simulink model "cf_compare_model"  (R2016a)
settings: Solver=FixedStepAuto  StartTime=0.0  StopTime=50  FixedStep=dt  RelTol=1e-3
values from neighbouring files (symbols this model uses):
  circ_amp = 3    [cf_pid_compare.m]
  circ_w = k    (= 0.666666666667)    [cf_pid_compare.m]
  ic = [-3 0 0 0 0 0 0 0 0 0 0 0]    [cf_pid_compare.m]    (also in main.m = [0 0 0 0 0 0 0 0 0 0 0 0])
  r2d = 180/pi    (= 57.2957795131)    [main.m]
  x_init = 0.0    (= 0)    [cf_pid_compare.m]
  x_vel = 1.0    (= 1)    [cf_pid_compare.m]
undefined symbols (not defined in the file or in its folder): default_ctl, est, geometric_ctl, pid_ctl
undefined symbols (not defined in the file): cf2
libraries: simulink x18, vrlib x12, aerolibtransform2 x12, cstblocks x8, aerolibutil x6, aerolibnav x3, dspmathops x2
(part 2 of 2)

== system cf_compare_model/Vehicle1/PWM 2 Speed ==
  PWM : Inport
  Add{,1..3} (4 alike) : Sum
  Constant{,1..3} (4 alike) : Constant  Value=model.pwm_offset
  Demux : Demux
  Gain{,1..3} (4 alike) : Gain  Gain=model.pwm_gain
  Mux : Mux
  Omega : Outport
  wires:
  Add3/1 -> Mux/4
  Demux/4 -> Gain3/1
  Add2/1 -> Mux/3
  Demux/3 -> Gain2/1
  Add1/1 -> Mux/2
  Demux/2 -> Gain1/1
  Constant3/1 -> Add3/1
  Gain3/1 -> Add3/2
  Constant2/1 -> Add2/1
  Gain2/1 -> Add2/2
  Constant1/1 -> Add1/1
  Gain1/1 -> Add1/2
  Add/1 -> Mux/1
  Demux/1 -> Gain/1
  Mux/1 -> Omega/1
  PWM/1 -> Demux/1
  Constant/1 -> Add/1
  Gain/1 -> Add/2

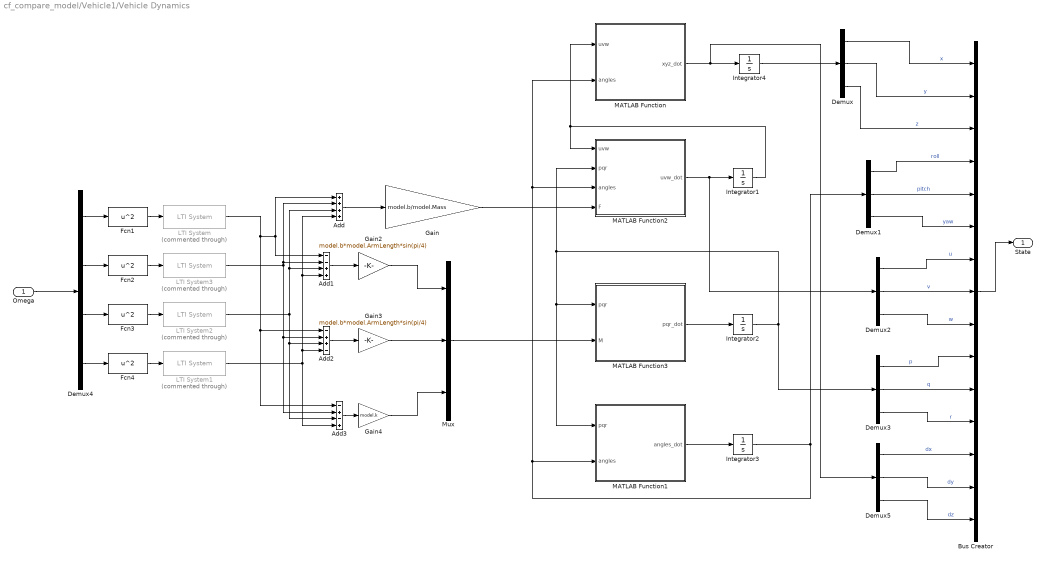
== system cf_compare_model/Vehicle1/Vehicle Dynamics ==
  Omega : Inport
  Add : Sum  Inputs=++++
  Add1 : Sum  Inputs=--++
  Add2 : Sum  Inputs=-++-
  Add3 : Sum  Inputs=-+-+
  Bus Creator : BusCreator  Inputs='x','y','z','roll','pitch','yaw','u','v','w','p','q','r','dx','dy','dz'
  Demux{,1..3,5} (5 alike) : Demux  Outputs=3
  Demux4 : Demux
  Fcn{1..4} (4 alike) : Fcn  Expr=u^2
  Gain : Gain  Gain=model.b/model.Mass
  Gain2 : Gain  Gain=model.b*model.ArmLength*sin(pi/4)
  Gain3 : Gain  Gain=model.b*model.ArmLength*sin(pi/4)
  Gain4 : Gain  Gain=model.k
  Integrator1 : Integrator  InitialCondition=ic(7:9)
  Integrator2 : Integrator  InitialCondition=ic(10:12)
  Integrator3 : Integrator  InitialCondition=ic(4:6)
  Integrator4 : Integrator  InitialCondition=ic(1:3)
  LTI System{,1..3} (4 alike) : cstblocks/LTI System  Commented=through  sys=model.motorDyn  IC=[]
  MATLAB Function : MATLAB Function  TreatAsAtomicUnit=on
  MATLAB Function1 : MATLAB Function  TreatAsAtomicUnit=on
  MATLAB Function2 : MATLAB Function  TreatAsAtomicUnit=on
  MATLAB Function3 : MATLAB Function  TreatAsAtomicUnit=on
  Mux : Mux  Inputs=3
  State : Outport
  wires:
  Omega/1 -> Demux4/1
  Demux4/4 -> Fcn4/1
  Demux4/3 -> Fcn3/1
  Demux4/2 -> Fcn2/1
  Demux4/1 -> Fcn1/1
  Demux2/2 -> Bus Creator/8  "v"
  Demux1/2 -> Bus Creator/5  "pitch"
  Demux3/1 -> Bus Creator/10  "p"
  Demux3/2 -> Bus Creator/11  "q"
  Demux3/3 -> Bus Creator/12  "r"
  Demux2/3 -> Bus Creator/9  "w"
  Demux2/1 -> Bus Creator/7  "u"
  Demux1/1 -> Bus Creator/4  "roll"
  Demux1/3 -> Bus Creator/6  "yaw"
  Demux/3 -> Bus Creator/3  "z"
  Demux/2 -> Bus Creator/2  "y"
  Demux/1 -> Bus Creator/1  "x"
  Integrator4/1 -> Demux/1
  Integrator2/1 -> MATLAB Function3/1(pqr), MATLAB Function1/1(pqr), MATLAB Function2/2(pqr), Demux3/1
  Integrator1/1 -> MATLAB Function2/1(uvw), MATLAB Function/1(uvw)
  Integrator3/1 -> MATLAB Function1/2(angles), MATLAB Function2/3(angles), MATLAB Function/2(angles), Demux1/1
  MATLAB Function1/1(angles_dot) -> Integrator3/1
  MATLAB Function3/1(pqr_dot) -> Integrator2/1
  MATLAB Function2/1(uvw_dot) -> Demux2/1, Integrator1/1
  MATLAB Function/1(xyz_dot) -> Integrator4/1, Demux5/1
  Mux/1 -> MATLAB Function3/2(M)
  Gain/1 -> MATLAB Function2/4(F)
  Gain3/1 -> Mux/2
  Add3/1 -> Gain4/1
  Gain4/1 -> Mux/3
  Gain2/1 -> Mux/1
  Add2/1 -> Gain3/1
  Add1/1 -> Gain2/1
  Bus Creator/1 -> State/1
  Fcn1/1 -> LTI System/1
  Fcn2/1 -> LTI System3/1
  Fcn3/1 -> LTI System2/1
  Fcn4/1 -> LTI System1/1
  Add/1 -> Gain/1
  LTI System1/1 -> Add3/4, Add2/4, Add1/4, Add/4
  LTI System2/1 -> Add3/3, Add2/3, Add/3, Add1/3
  LTI System3/1 -> Add3/2, Add2/2, Add/2, Add1/2
  LTI System/1 -> Add3/1, Add2/1, Add1/1, Add/1
  Demux5/1 -> Bus Creator/13  "dx"
  Demux5/2 -> Bus Creator/14  "dy"
  Demux5/3 -> Bus Creator/15  "dz"

== system cf_compare_model/Vehicle3/PWM 2 Speed ==
  PWM : Inport
  Add{,1..3} (4 alike) : Sum
  Constant{,1..3} (4 alike) : Constant  Value=model.pwm_offset
  Demux : Demux
  Gain{,1..3} (4 alike) : Gain  Gain=model.pwm_gain
  Mux : Mux
  Omega : Outport
  wires:
  Add3/1 -> Mux/4
  Demux/4 -> Gain3/1
  Add2/1 -> Mux/3
  Demux/3 -> Gain2/1
  Add1/1 -> Mux/2
  Demux/2 -> Gain1/1
  Constant3/1 -> Add3/1
  Gain3/1 -> Add3/2
  Constant2/1 -> Add2/1
  Gain2/1 -> Add2/2
  Constant1/1 -> Add1/1
  Gain1/1 -> Add1/2
  Add/1 -> Mux/1
  Demux/1 -> Gain/1
  Mux/1 -> Omega/1
  PWM/1 -> Demux/1
  Constant/1 -> Add/1
  Gain/1 -> Add/2

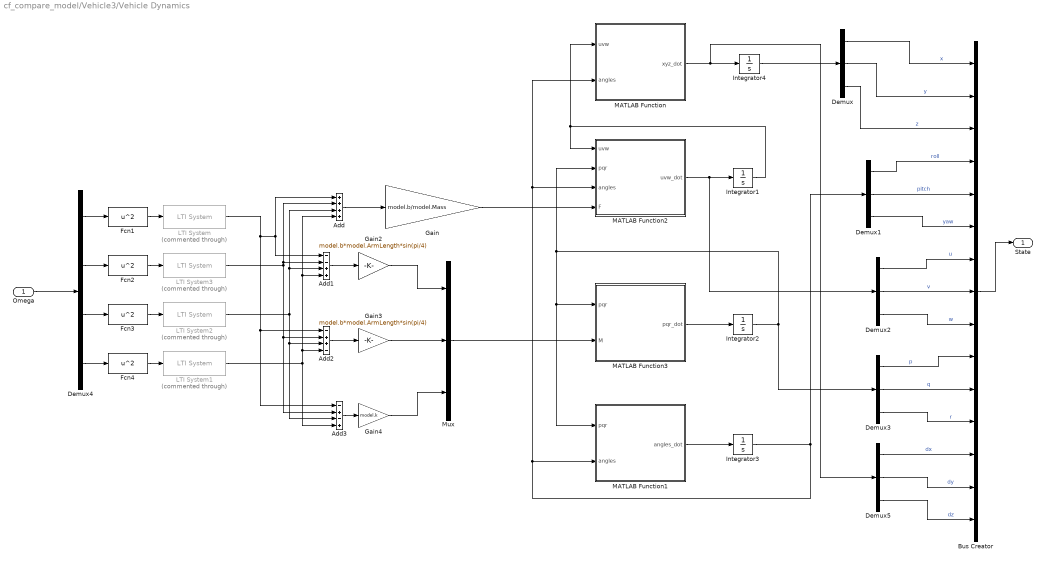
== system cf_compare_model/Vehicle3/Vehicle Dynamics ==
  Omega : Inport
  Add : Sum  Inputs=++++
  Add1 : Sum  Inputs=--++
  Add2 : Sum  Inputs=-++-
  Add3 : Sum  Inputs=-+-+
  Bus Creator : BusCreator  Inputs='x','y','z','roll','pitch','yaw','u','v','w','p','q','r','dx','dy','dz'
  Demux{,1..3,5} (5 alike) : Demux  Outputs=3
  Demux4 : Demux
  Fcn{1..4} (4 alike) : Fcn  Expr=u^2
  Gain : Gain  Gain=model.b/model.Mass
  Gain2 : Gain  Gain=model.b*model.ArmLength*sin(pi/4)
  Gain3 : Gain  Gain=model.b*model.ArmLength*sin(pi/4)
  Gain4 : Gain  Gain=model.k
  Integrator1 : Integrator  InitialCondition=ic(7:9)
  Integrator2 : Integrator  InitialCondition=ic(10:12)
  Integrator3 : Integrator  InitialCondition=ic(4:6)
  Integrator4 : Integrator  InitialCondition=ic(1:3)
  LTI System{,1..3} (4 alike) : cstblocks/LTI System  Commented=through  sys=model.motorDyn  IC=[]
  MATLAB Function : MATLAB Function  TreatAsAtomicUnit=on
  MATLAB Function1 : MATLAB Function  TreatAsAtomicUnit=on
  MATLAB Function2 : MATLAB Function  TreatAsAtomicUnit=on
  MATLAB Function3 : MATLAB Function  TreatAsAtomicUnit=on
  Mux : Mux  Inputs=3
  State : Outport
  wires:
  Omega/1 -> Demux4/1
  Demux4/4 -> Fcn4/1
  Demux4/3 -> Fcn3/1
  Demux4/2 -> Fcn2/1
  Demux4/1 -> Fcn1/1
  Demux2/2 -> Bus Creator/8  "v"
  Demux1/2 -> Bus Creator/5  "pitch"
  Demux3/1 -> Bus Creator/10  "p"
  Demux3/2 -> Bus Creator/11  "q"
  Demux3/3 -> Bus Creator/12  "r"
  Demux2/3 -> Bus Creator/9  "w"
  Demux2/1 -> Bus Creator/7  "u"
  Demux1/1 -> Bus Creator/4  "roll"
  Demux1/3 -> Bus Creator/6  "yaw"
  Demux/3 -> Bus Creator/3  "z"
  Demux/2 -> Bus Creator/2  "y"
  Demux/1 -> Bus Creator/1  "x"
  Integrator4/1 -> Demux/1
  Integrator2/1 -> MATLAB Function3/1(pqr), MATLAB Function1/1(pqr), MATLAB Function2/2(pqr), Demux3/1
  Integrator1/1 -> MATLAB Function2/1(uvw), MATLAB Function/1(uvw)
  Integrator3/1 -> MATLAB Function1/2(angles), MATLAB Function2/3(angles), MATLAB Function/2(angles), Demux1/1
  MATLAB Function1/1(angles_dot) -> Integrator3/1
  MATLAB Function3/1(pqr_dot) -> Integrator2/1
  MATLAB Function2/1(uvw_dot) -> Demux2/1, Integrator1/1
  MATLAB Function/1(xyz_dot) -> Integrator4/1, Demux5/1
  Mux/1 -> MATLAB Function3/2(M)
  Gain/1 -> MATLAB Function2/4(F)
  Gain3/1 -> Mux/2
  Add3/1 -> Gain4/1
  Gain4/1 -> Mux/3
  Gain2/1 -> Mux/1
  Add2/1 -> Gain3/1
  Add1/1 -> Gain2/1
  Bus Creator/1 -> State/1
  Fcn1/1 -> LTI System/1
  Fcn2/1 -> LTI System3/1
  Fcn3/1 -> LTI System2/1
  Fcn4/1 -> LTI System1/1
  Add/1 -> Gain/1
  LTI System1/1 -> Add3/4, Add2/4, Add1/4, Add/4
  LTI System2/1 -> Add3/3, Add2/3, Add/3, Add1/3
  LTI System3/1 -> Add3/2, Add2/2, Add/2, Add1/2
  LTI System/1 -> Add3/1, Add2/1, Add1/1, Add/1
  Demux5/1 -> Bus Creator/13  "dx"
  Demux5/2 -> Bus Creator/14  "dy"
  Demux5/3 -> Bus Creator/15  "dz"

== system cf_compare_model/circle xy/acc_circ ==
  Constant : Constant  Value=0
  Mux : Mux  Inputs=3
  Sine Wave1 : Sin  Amplitude=circ_amp*circ_w^2  Frequency=circ_w  Phase=3*pi/2  SampleTime=0
  Sine Wave2 : Sin  Amplitude=circ_amp*circ_w^2  Frequency=circ_w  Phase=pi  SampleTime=0
  Acc : Outport
  wires:
  Sine Wave2/1 -> Mux/3
  Constant/1 -> Mux/1
  Sine Wave1/1 -> Mux/2
  Mux/1 -> Acc/1

== system cf_compare_model/circle xy/jerk_circ ==
  Constant : Constant  Value=0
  Mux : Mux  Inputs=3
  Sine Wave1 : Sin  Amplitude=circ_amp*circ_w^3  Frequency=circ_w  SampleTime=0
  Sine Wave2 : Sin  Amplitude=circ_amp*circ_w^3  Frequency=circ_w  Phase=3*pi/2  SampleTime=0
  Jerk : Outport
  wires:
  Sine Wave2/1 -> Mux/3
  Constant/1 -> Mux/1
  Sine Wave1/1 -> Mux/2
  Mux/1 -> Jerk/1

== system cf_compare_model/circle xy/snap_circ ==
  Constant : Constant  Value=0
  Mux : Mux  Inputs=3
  Sine Wave1 : Sin  Amplitude=circ_amp*circ_w^4  Frequency=circ_w  Phase=pi/2  SampleTime=0
  Sine Wave2 : Sin  Amplitude=circ_amp*circ_w^4  Frequency=circ_w  SampleTime=0
  Snap : Outport
  wires:
  Sine Wave2/1 -> Mux/3
  Constant/1 -> Mux/1
  Sine Wave1/1 -> Mux/2
  Mux/1 -> Snap/1

== system cf_compare_model/circle xy/vel_circ ==
  Constant : Constant  Value=x_vel
  Mux : Mux  Inputs=3
  Sine Wave1 : Sin  Amplitude=circ_amp*circ_w  Frequency=circ_w  Phase=pi  SampleTime=0
  Sine Wave2 : Sin  Amplitude=circ_amp*circ_w  Frequency=circ_w  Phase=pi/2  SampleTime=0
  Vel : Outport
  wires:
  Sine Wave2/1 -> Mux/3
  Constant/1 -> Mux/1
  Sine Wave1/1 -> Mux/2
  Mux/1 -> Vel/1

== system cf_compare_model/circle yz /acc_circ ==
  Constant : Constant  Value=0
  Mux : Mux  Inputs=3
  Sine Wave1 : Sin  Amplitude=circ_amp*circ_w^2  Frequency=circ_w  Phase=3*pi/2  SampleTime=0
  Sine Wave2 : Sin  Amplitude=circ_amp*circ_w^2  Frequency=circ_w  Phase=pi  SampleTime=0
  Acc : Outport
  wires:
  Sine Wave2/1 -> Mux/3
  Constant/1 -> Mux/1
  Sine Wave1/1 -> Mux/2
  Mux/1 -> Acc/1

== system cf_compare_model/circle yz /jerk_circ ==
  Constant : Constant  Value=0
  Mux : Mux  Inputs=3
  Sine Wave1 : Sin  Amplitude=circ_amp*circ_w^3  Frequency=circ_w  SampleTime=0
  Sine Wave2 : Sin  Amplitude=circ_amp*circ_w^3  Frequency=circ_w  Phase=3*pi/2  SampleTime=0
  Jerk : Outport
  wires:
  Sine Wave2/1 -> Mux/3
  Constant/1 -> Mux/1
  Sine Wave1/1 -> Mux/2
  Mux/1 -> Jerk/1

== system cf_compare_model/circle yz /snap_circ ==
  Constant : Constant  Value=0
  Mux : Mux  Inputs=3
  Sine Wave1 : Sin  Amplitude=circ_amp*circ_w^4  Frequency=circ_w  Phase=pi/2  SampleTime=0
  Sine Wave2 : Sin  Amplitude=circ_amp*circ_w^4  Frequency=circ_w  SampleTime=0
  Snap : Outport
  wires:
  Sine Wave2/1 -> Mux/3
  Constant/1 -> Mux/1
  Sine Wave1/1 -> Mux/2
  Mux/1 -> Snap/1

== system cf_compare_model/circle yz /vel_circ ==
  Constant : Constant  Value=x_vel
  Mux : Mux  Inputs=3
  Sine Wave1 : Sin  Amplitude=circ_amp*circ_w  Frequency=circ_w  Phase=pi  SampleTime=0
  Sine Wave2 : Sin  Amplitude=circ_amp*circ_w  Frequency=circ_w  Phase=pi/2  SampleTime=0
  Vel : Outport
  wires:
  Sine Wave2/1 -> Mux/3
  Constant/1 -> Mux/1
  Sine Wave1/1 -> Mux/2
  Mux/1 -> Vel/1

== system cf_compare_model/PID/Estimator/AddNoise1 ==
  Signal : Inport
  AddNoise : Subsystem
  AddNoise1 : Subsystem
  AddNoise2 : Subsystem
  Demux : Demux  Outputs=3
  Mux : Mux  Inputs=3
  +Noise : Outport
  wires:
  Mux/1 -> +Noise/1
  Signal/1 -> Demux/1
  AddNoise2/1(+Noise) -> Mux/3
  AddNoise1/1(+Noise) -> Mux/2
  AddNoise/1(+Noise) -> Mux/1
  Demux/1 -> AddNoise/1(Signal)
  Demux/3 -> AddNoise2/1(Signal)
  Demux/2 -> AddNoise1/1(Signal)

== system cf_compare_model/PID/Estimator/AddNoise3 ==
  Signal : Inport
  AddNoise : Subsystem
  AddNoise1 : Subsystem
  AddNoise2 : Subsystem
  Demux : Demux  Outputs=3
  Mux : Mux  Inputs=3
  +Noise : Outport
  wires:
  Demux/2 -> AddNoise1/1(Signal)
  Demux/3 -> AddNoise2/1(Signal)
  Demux/1 -> AddNoise/1(Signal)
  AddNoise/1(+Noise) -> Mux/1
  AddNoise1/1(+Noise) -> Mux/2
  AddNoise2/1(+Noise) -> Mux/3
  Signal/1 -> Demux/1
  Mux/1 -> +Noise/1

== system cf_compare_model/PID/Estimator/Mahoney ==
  A : Inport  PortDimensions=[1 3]
  ω : Inport  Port=2  PortDimensions=[1 3]
  Vicon : Inport  Port=3
  q : Inport  Port=4  PortDimensions=[1 4]
  Acceleration Error Estimate : Scope
  Add : Sum  Inputs=+++
  Add1 : Sum
  Constant : Constant  Value=0
  Cross Product : vrlib/Utilities/Cross Product
  Cross Product1 : vrlib/Utilities/Cross Product
  Gain1 : Gain  Gain=0.5
  Integrator : Integrator
  Integrator1 : Integrator  InitialCondition=[1,0,0,0]
  Ki : Gain  Gain=est.Ki
  Kp : Gain  Gain=est.Kp
  Mux : Mux  Inputs=2
  Normalize Vector : vrlib/Utilities/Normalize Vector  maxzero=.01
  Normalize Vector1 : vrlib/Utilities/Normalize Vector  maxzero=10e-4
  Total Error Estimate : Scope
  Vicon Error Estimate : Scope
  calc v : MATLAB Function  TreatAsAtomicUnit=on
  calc v3 : MATLAB Function  TreatAsAtomicUnit=on
  quatprod : MATLAB Function  TreatAsAtomicUnit=on
  Quaternion : Outport
  wires:
  A/1 -> Normalize Vector/1
  Constant/1 -> Mux/1
  Add1/1 -> Integrator/1, Kp/1, Total Error Estimate/1
  Ki/1 -> Add/2
  calc v/1(v) -> Cross Product/1, Cross Product1/2
  Add/1 -> Mux/2
  Kp/1 -> Add/1
  Gain1/1 -> Integrator1/1
  quatprod/1(ab) -> Gain1/1
  Mux/1 -> quatprod/2(b)
  Integrator/1 -> Ki/1
  Integrator1/1 -> Normalize Vector1/1
  Normalize Vector1/1 -> Quaternion/1
  q/1 -> calc v/1(q), quatprod/1(a)
  Cross Product/1 -> Acceleration Error Estimate/1, Add1/2
  Vicon/1 -> calc v3/1(q)
  Cross Product1/1 -> Vicon Error Estimate/1, Add1/1
  calc v3/1(v) -> Cross Product1/1
  Normalize Vector/1 -> Cross Product/2
  ω/1 -> Add/3

== system cf_compare_model/PID/PID Controller/Attitude Control ==
  desired_attitude : Inport
  attitutde : Inport  Port=2
  Demux : Demux  Outputs=3
  Demux1 : Demux  Outputs=3
  Gain : Gain  Gain=r2d
  Gain1 : Gain  Gain=r2d
  Gain2 : Gain  Gain=r2d
  Mux : Mux  Inputs=3
  PID : Subsystem
  PID1 : Subsystem
  PID2 : Subsystem
  Saturation : Saturate  UpperLimit=sat(3)  LowerLimit=-sat(3)
  Saturation1 : Saturate  UpperLimit=sat(2)  LowerLimit=-sat(2)
  Saturation2 : Saturate  UpperLimit=sat(1)  LowerLimit=-sat(1)
  desired_rates : Outport
  wires:
  [pitch] -> PID1/2(Measured)
  [desired_pitch] -> PID1/1(Desired)
  [desired_roll] -> PID/1(Desired)
  [roll] -> PID/2(Measured)
  desired_attitude/1 -> Demux/1
  Demux/1 -> Saturation2/1
  Demux/2 -> Saturation1/1
  Demux/3 -> [desired_yaw]
  attitutde/1 -> Demux1/1
  Demux1/1 -> Gain/1
  Demux1/2 -> Gain1/1
  Demux1/3 -> Gain2/1
  [yaw] -> PID2/2(Measured)
  Gain/1 -> [roll]
  Gain1/1 -> [pitch]
  Gain2/1 -> [yaw]
  [desired_yaw] -> PID2/1(Desired)
  PID/1(Output) -> Mux/1
  PID2/1(Output) -> Saturation/1
  PID1/1(Output) -> Mux/2
  Mux/1 -> desired_rates/1
  Saturation/1 -> Mux/3
  Saturation1/1 -> [desired_pitch]
  Saturation2/1 -> [desired_roll]

== system cf_compare_model/PID/PID Controller/Linear Velocity Control ==
  note: ROLL CONTROLS Y TRANSLATION
  note: PITCH CONTROLS X TRANSLATION
  position_error : Inport
  velocity : Inport  Port=2
  Add : Sum
  Demux : Demux  Outputs=3
  Demux1 : Demux  Outputs=3
  "Min_thrust " : Constant  Value=default_ctl.pwm  SampleTime=0
  Mux : Mux  Inputs=2
  PID : Subsystem
  PID1 : Subsystem
  PID_Altitude : Subsystem
  Saturation2 : Saturate  UpperLimit=default_ctl.sat(4,1)  LowerLimit=0
  Scope : Scope
  Terminator : Terminator
  desired_attitude : Outport
  desired_thrust : Outport  Port=2
  wires:
  [y_e] -> PID/1(Desired)
  Saturation2/1 -> Scope/1, desired_thrust/1
  "Min_thrust "/1 -> Add/2
  Add/1 -> Saturation2/1
  PID_Altitude/1(Adjust) -> Add/1
  position_error/1 -> Demux/1
  Demux/1 -> [x_e]
  Demux/2 -> [y_e]
  Demux/3 -> [z_e]
  [z_e] -> PID_Altitude/1(z_error)
  velocity/1 -> Demux1/1
  Demux1/1 -> [v_x]
  Demux1/2 -> [v_y]
  Demux1/3 -> Terminator/1
  [v_y] -> PID/2(Measured)
  Mux/1 -> desired_attitude/1
  PID/1(Output) -> Mux/1
  [x_e] -> PID1/1(Desired)
  [v_x] -> PID1/2(Measured)
  PID1/1(Output) -> Mux/2

== system cf_compare_model/PID/PID Controller/Motor Mix ==
  rpy : Inport
  T : Inport  Port=2
  Constant : Constant  Value=mix
  Demux : Demux  Outputs=3
  Mux : Mux
  Product : Product  Multiplication=Matrix(*)
  PWM : Outport
  wires:
  T/1 -> Mux/4
  Mux/1 -> Product/2
  Product/1 -> PWM/1
  Constant/1 -> Product/1
  rpy/1 -> Demux/1
  Demux/2 -> Mux/2
  Demux/1 -> Mux/1
  Demux/3 -> Mux/3

== system cf_compare_model/PID/PID Controller/Rate Control ==
  note: roll
      | pitch
      | yaw
  desired_rates : Inport
  rates : Inport  Port=2
  Demux : Demux  Outputs=3
  Demux1 : Demux  Outputs=3
  Gain : Gain  Gain=r2d
  Gain1 : Gain  Gain=r2d
  Gain2 : Gain  Gain=r2d
  Mux : Mux  Inputs=3
  PID : Subsystem
  PID1 : Subsystem
  PID2 : Subsystem
  rpy_cmd : Outport
  wires:
  desired_rates/1 -> Demux/1
  Demux/1 -> [desired_droll]
  Demux/2 -> [desired_dpitch]
  Demux/3 -> [desired_dyaw]
  rates/1 -> Demux1/1
  Demux1/1 -> Gain/1
  Demux1/2 -> Gain1/1
  Demux1/3 -> Gain2/1
  Gain/1 -> [droll]
  Gain1/1 -> [dpitch]
  Gain2/1 -> [dyaw]
  PID2/1(Output) -> Mux/3
  PID1/1(Output) -> Mux/2
  PID/1(Output) -> Mux/1
  Mux/1 -> rpy_cmd/1
  [desired_dyaw] -> PID2/1(Desired)
  [desired_droll] -> PID/1(Desired)
  [desired_dpitch] -> PID1/1(Desired)
  [dpitch] -> PID1/2(Measured)
  [droll] -> PID/2(Measured)
  [dyaw] -> PID2/2(Measured)

== system cf_compare_model/PID/Vehicle/PWM 2 Speed ==
  PWM : Inport
  Add{,1..3} (4 alike) : Sum
  Constant{,1..3} (4 alike) : Constant  Value=model.pwm_offset
  Demux : Demux
  Gain{,1..3} (4 alike) : Gain  Gain=model.pwm_gain
  Mux : Mux
  Omega : Outport
  wires:
  Gain/1 -> Add/2
  Constant/1 -> Add/1
  PWM/1 -> Demux/1
  Mux/1 -> Omega/1
  Demux/1 -> Gain/1
  Add/1 -> Mux/1
  Gain1/1 -> Add1/2
  Constant1/1 -> Add1/1
  Gain2/1 -> Add2/2
  Constant2/1 -> Add2/1
  Gain3/1 -> Add3/2
  Constant3/1 -> Add3/1
  Demux/2 -> Gain1/1
  Add1/1 -> Mux/2
  Demux/3 -> Gain2/1
  Add2/1 -> Mux/3
  Demux/4 -> Gain3/1
  Add3/1 -> Mux/4

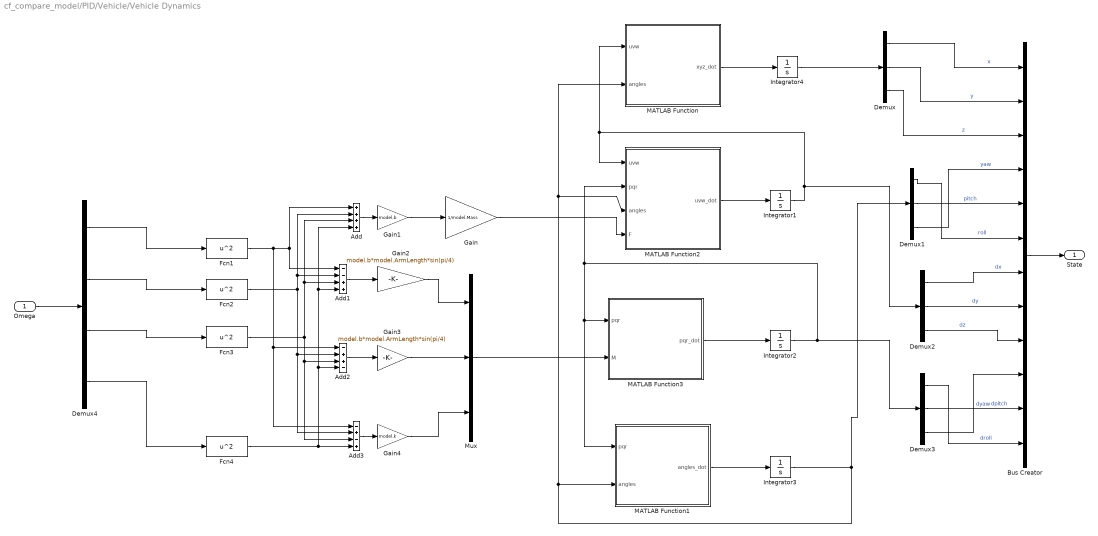
== system cf_compare_model/PID/Vehicle/Vehicle Dynamics ==
  Omega : Inport
  Add : Sum  Inputs=++++
  Add1 : Sum  Inputs=--++
  Add2 : Sum  Inputs=-++-
  Add3 : Sum  Inputs=-+-+
  Bus Creator : BusCreator  Inputs=12
  Demux{,1..3} (4 alike) : Demux  Outputs=3
  Demux4 : Demux
  Fcn{1..4} (4 alike) : Fcn  Expr=u^2
  Gain : Gain  Gain=1/model.Mass
  Gain1 : Gain  Gain=model.b
  Gain2 : Gain  Gain=model.b*model.ArmLength*sin(pi/4)
  Gain3 : Gain  Gain=model.b*model.ArmLength*sin(pi/4)
  Gain4 : Gain  Gain=model.k
  Integrator1 : Integrator  InitialCondition=ic(7:9)
  Integrator2 : Integrator  InitialCondition=ic(10:12)
  Integrator3 : Integrator  InitialCondition=ic(4:6)
  Integrator4 : Integrator  InitialCondition=ic(1:3)
  MATLAB Function : MATLAB Function  TreatAsAtomicUnit=on
  MATLAB Function1 : MATLAB Function  TreatAsAtomicUnit=on
  MATLAB Function2 : MATLAB Function  TreatAsAtomicUnit=on
  MATLAB Function3 : MATLAB Function  TreatAsAtomicUnit=on
  Mux : Mux  Inputs=3
  State : Outport
  wires:
  Gain1/1 -> Gain/1
  Fcn4/1 -> Add/4, Add1/4, Add2/4, Add3/4
  Fcn3/1 -> Add1/3, Add/3, Add2/3, Add3/3
  Fcn2/1 -> Add2/2, Add3/2, Add1/2, Add/2
  Fcn1/1 -> Add/1, Add1/1, Add2/1, Add3/1
  Bus Creator/1 -> State/1
  Add1/1 -> Gain2/1
  Add/1 -> Gain1/1
  Add2/1 -> Gain3/1
  Gain2/1 -> Mux/1
  Gain4/1 -> Mux/3
  Add3/1 -> Gain4/1
  Gain3/1 -> Mux/2
  Gain/1 -> MATLAB Function2/4(F)
  Mux/1 -> MATLAB Function3/2(M)
  MATLAB Function/1(xyz_dot) -> Integrator4/1
  MATLAB Function2/1(uvw_dot) -> Integrator1/1
  MATLAB Function3/1(pqr_dot) -> Integrator2/1
  MATLAB Function1/1(angles_dot) -> Integrator3/1
  Integrator3/1 -> Demux1/1, MATLAB Function/2(angles), MATLAB Function2/3(angles), MATLAB Function1/2(angles)
  Integrator1/1 -> Demux2/1, MATLAB Function/1(uvw), MATLAB Function2/1(uvw)
  Integrator2/1 -> Demux3/1, MATLAB Function2/2(pqr), MATLAB Function1/1(pqr), MATLAB Function3/1(pqr)
  Integrator4/1 -> Demux/1
  Demux/1 -> Bus Creator/1  "x"
  Demux/2 -> Bus Creator/2  "y"
  Demux/3 -> Bus Creator/3  "z"
  Demux1/3 -> Bus Creator/4  "yaw"
  Demux1/1 -> Bus Creator/6  "roll"
  Demux2/1 -> Bus Creator/7  "dx"
  Demux2/3 -> Bus Creator/9  "dz"
  Demux3/3 -> Bus Creator/10  "dyaw"
  Demux3/2 -> Bus Creator/11  "dpitch"
  Demux3/1 -> Bus Creator/12  "droll"
  Demux1/2 -> Bus Creator/5  "pitch"
  Demux2/2 -> Bus Creator/8  "dy"
  Demux4/1 -> Fcn1/1
  Demux4/2 -> Fcn2/1
  Demux4/3 -> Fcn3/1
  Demux4/4 -> Fcn4/1
  Omega/1 -> Demux4/1

== system cf_compare_model/PID Controller/Attitude Control/PID ==
  Desired : Inport
  Measured : Inport  Port=2
  Add : Sum  Inputs=3
  Derivative : Derivative
  Integrator Limited : Integrator  LimitOutput=on  UpperSaturationLimit=intSat(2,1)  LowerSaturationLimit=-intSat(2,1)
  Kd : Gain  Gain=att(1,3)  OutMin=[-200]  OutMax=[200]
  Ki : Gain  Gain=att(1,2)  OutMin=[-200]  OutMax=[200]
  Kp : Gain  Gain=att(1,1)  OutMin=[-200]  OutMax=[200]
  Subtract : Sum  Inputs=+-
  Output : Outport
  wires:
  Measured/1 -> Subtract/2
  Desired/1 -> Subtract/1
  Ki/1 -> Add/2
  Add/1 -> Output/1
  Kp/1 -> Add/1
  Kd/1 -> Add/3
  Subtract/1 -> Kp/1, Integrator Limited/1, Derivative/1
  Integrator Limited/1 -> Ki/1
  Derivative/1 -> Kd/1

== system cf_compare_model/PID Controller/Attitude Control/PID1 ==
  Desired : Inport
  Measured : Inport  Port=2
  Add : Sum  Inputs=3
  Derivative : Derivative
  Integrator Limited1 : Integrator  LimitOutput=on  UpperSaturationLimit=intSat(2,2)  LowerSaturationLimit=-intSat(2,2)
  Kd : Gain  Gain=att(2,3)  OutMin=[-200]  OutMax=[200]
  Ki : Gain  Gain=att(2,2)  OutMin=[-200]  OutMax=[200]
  Kp : Gain  Gain=att(2,1)  OutMin=[-200]  OutMax=[200]
  Subtract : Sum  Inputs=+-
  Output : Outport
  wires:
  Derivative/1 -> Kd/1
  Integrator Limited1/1 -> Ki/1
  Subtract/1 -> Integrator Limited1/1, Derivative/1, Kp/1
  Kd/1 -> Add/3
  Kp/1 -> Add/1
  Add/1 -> Output/1
  Ki/1 -> Add/2
  Desired/1 -> Subtract/1
  Measured/1 -> Subtract/2

== system cf_compare_model/PID Controller/Attitude Control/PID2 ==
  Desired : Inport
  Measured : Inport  Port=2
  Add : Sum  Inputs=3
  Derivative : Derivative
  Integrator Limited : Integrator  LimitOutput=on  UpperSaturationLimit=intSat(2,3)  LowerSaturationLimit=-intSat(2,3)
  Kd : Gain  Gain=att(3,3)  OutMin=[-200]  OutMax=[200]
  Ki : Gain  Gain=att(3,2)  OutMin=[-200]  OutMax=[200]
  Kp : Gain  Gain=att(3,1)  OutMin=[-200]  OutMax=[200]
  Subtract : Sum  Inputs=+-
  Output : Outport
  wires:
  Measured/1 -> Subtract/2
  Desired/1 -> Subtract/1
  Ki/1 -> Add/2
  Add/1 -> Output/1
  Kp/1 -> Add/1
  Kd/1 -> Add/3
  Subtract/1 -> Kp/1, Integrator Limited/1, Derivative/1
  Integrator Limited/1 -> Ki/1
  Derivative/1 -> Kd/1

== system cf_compare_model/PID Controller/Linear Velocity Control/PID ==
  Desired : Inport
  Measured : Inport  Port=2
  Add : Sum  Inputs=3
  Derivative : Derivative
  Integrator Limited : Integrator  LimitOutput=on  UpperSaturationLimit=intSat(1,1)  LowerSaturationLimit=-intSat(1,1)
  Kd : Gain  Gain=pos(1,3)  OutMin=[-200]  OutMax=[200]
  Ki : Gain  Gain=pos(1,2)  OutMin=[-200]  OutMax=[200]
  Kp : Gain  Gain=pos(1,1)  OutMin=[-200]  OutMax=[200]
  Subtract : Sum  Inputs=+-
  Output : Outport
  wires:
  Measured/1 -> Subtract/2
  Desired/1 -> Subtract/1
  Ki/1 -> Add/2
  Add/1 -> Output/1
  Kp/1 -> Add/1
  Kd/1 -> Add/3
  Subtract/1 -> Kp/1, Integrator Limited/1, Derivative/1
  Integrator Limited/1 -> Ki/1
  Derivative/1 -> Kd/1

== system cf_compare_model/PID Controller/Linear Velocity Control/PID1 ==
  Desired : Inport
  Measured : Inport  Port=2
  Add : Sum  Inputs=3
  Derivative : Derivative
  Integrator Limited : Integrator  LimitOutput=on  UpperSaturationLimit=intSat(1,2)  LowerSaturationLimit=-intSat(1,2)
  Kd : Gain  Gain=pos(2,3)  OutMin=[-200]  OutMax=[200]
  Ki : Gain  Gain=pos(2,2)  OutMin=[-200]  OutMax=[200]
  Kp : Gain  Gain=pos(2,1)  OutMin=[-200]  OutMax=[200]
  Subtract : Sum  Inputs=+-
  Output : Outport
  wires:
  Derivative/1 -> Kd/1
  Integrator Limited/1 -> Ki/1
  Subtract/1 -> Derivative/1, Integrator Limited/1, Kp/1
  Kd/1 -> Add/3
  Kp/1 -> Add/1
  Add/1 -> Output/1
  Ki/1 -> Add/2
  Desired/1 -> Subtract/1
  Measured/1 -> Subtract/2

== system cf_compare_model/PID Controller/Linear Velocity Control/PID_Altitude ==
  z_error : Inport
  Add : Sum  Inputs=3
  Derivative : Derivative
  Integrator Limited : Integrator  LimitOutput=on  UpperSaturationLimit=1000  LowerSaturationLimit=-1000
  Kd : Gain  Gain=pos(3,3)  OutMin=[-200]  OutMax=[200]
  Ki : Gain  Gain=pos(3,2)  OutMin=[-200]  OutMax=[200]
  Kp : Gain  Gain=pos(3,1)  OutMin=[-200]  OutMax=[200]
  Adjust : Outport
  wires:
  Derivative/1 -> Kd/1
  Integrator Limited/1 -> Ki/1
  Kd/1 -> Add/3
  Kp/1 -> Add/1
  Ki/1 -> Add/2
  Add/1 -> Adjust/1
  z_error/1 -> Kp/1, Derivative/1, Integrator Limited/1

== system cf_compare_model/PID Controller/Linear Velocity Control/norm2 ==
  Vec : Inport
  Dot Product1 : DotProduct  InputSameDT=on  OutDataTypeStr=Inherit: Inherit via internal rule
  Math Function1 : Math  Operator=transpose  SaturateOnIntegerOverflow=on
  Sqrt : Sqrt  SaturateOnIntegerOverflow=on
  Norm : Outport
  wires:
  Vec/1 -> Math Function1/1, Dot Product1/1
  Dot Product1/1 -> Sqrt/1
  Math Function1/1 -> Dot Product1/2
  Sqrt/1 -> Norm/1

== system cf_compare_model/PID Controller/Rate Control/PID ==
  Desired : Inport
  Measured : Inport  Port=2
  Add : Sum  Inputs=3
  Derivative : Derivative
  Integrator Limited : Integrator  LimitOutput=on  UpperSaturationLimit=intSat(3,1)  LowerSaturationLimit=-intSat(3,1)
  Kd : Gain  Gain=rates(1,3)  OutMin=[-200]  OutMax=[200]
  Ki : Gain  Gain=rates(1,2)  OutMin=[-200]  OutMax=[200]
  Kp : Gain  Gain=rates(1,1)  OutMin=[-200]  OutMax=[200]
  Subtract : Sum  Inputs=+-
  Output : Outport
  wires:
  Measured/1 -> Subtract/2
  Desired/1 -> Subtract/1
  Ki/1 -> Add/2
  Add/1 -> Output/1
  Kp/1 -> Add/1
  Kd/1 -> Add/3
  Subtract/1 -> Kp/1, Integrator Limited/1, Derivative/1
  Integrator Limited/1 -> Ki/1
  Derivative/1 -> Kd/1

== system cf_compare_model/PID Controller/Rate Control/PID1 ==
  Desired : Inport
  Measured : Inport  Port=2
  Add : Sum  Inputs=3
  Derivative : Derivative
  Integrator Limited : Integrator  LimitOutput=on  UpperSaturationLimit=intSat(3,2)  LowerSaturationLimit=-intSat(3,2)
  Kd : Gain  Gain=rates(2,3)  OutMin=[-200]  OutMax=[200]
  Ki : Gain  Gain=rates(2,2)  OutMin=[-200]  OutMax=[200]
  Kp : Gain  Gain=rates(2,1)  OutMin=[-200]  OutMax=[200]
  Subtract : Sum  Inputs=+-
  Output : Outport
  wires:
  Derivative/1 -> Kd/1
  Integrator Limited/1 -> Ki/1
  Subtract/1 -> Derivative/1, Integrator Limited/1, Kp/1
  Kd/1 -> Add/3
  Kp/1 -> Add/1
  Add/1 -> Output/1
  Ki/1 -> Add/2
  Desired/1 -> Subtract/1
  Measured/1 -> Subtract/2

== system cf_compare_model/PID Controller/Rate Control/PID2 ==
  Desired : Inport
  Measured : Inport  Port=2
  Add : Sum  Inputs=3
  Derivative : Derivative
  Integrator Limited : Integrator  LimitOutput=on  UpperSaturationLimit=intSat(3,3)  LowerSaturationLimit=-intSat(3,3)
  Kd : Gain  Gain=rates(3,3)  OutMin=[-200]  OutMax=[200]
  Ki : Gain  Gain=rates(3,2)  OutMin=[-200]  OutMax=[200]
  Kp : Gain  Gain=rates(3,1)  OutMin=[-200]  OutMax=[200]
  Subtract : Sum  Inputs=+-
  Output : Outport
  wires:
  Measured/1 -> Subtract/2
  Desired/1 -> Subtract/1
  Ki/1 -> Add/2
  Add/1 -> Output/1
  Kp/1 -> Add/1
  Kd/1 -> Add/3
  Subtract/1 -> Kp/1, Integrator Limited/1, Derivative/1
  Integrator Limited/1 -> Ki/1
  Derivative/1 -> Kd/1

== system cf_compare_model/PID/Estimator/AddNoise1/AddNoise ==
  Signal : Inport
  Add2 : Sum
  Band-Limited White Noise : simulink/Sources/Band-Limited White Noise  Cov=0.00005  Ts=0.1  seed=rng_seed
  +Noise : Outport
  wires:
  Band-Limited White Noise/1 -> Add2/2
  Signal/1 -> Add2/1
  Add2/1 -> +Noise/1

== system cf_compare_model/PID/Estimator/AddNoise1/AddNoise1 ==
  Signal : Inport
  Add2 : Sum
  Band-Limited White Noise : simulink/Sources/Band-Limited White Noise  Cov=0.00005  Ts=0.1  seed=rng_seed
  +Noise : Outport
  wires:
  Add2/1 -> +Noise/1
  Signal/1 -> Add2/1
  Band-Limited White Noise/1 -> Add2/2

== system cf_compare_model/PID/Estimator/AddNoise1/AddNoise2 ==
  Signal : Inport
  Add2 : Sum
  Band-Limited White Noise : simulink/Sources/Band-Limited White Noise  Cov=0.00005  Ts=0.1  seed=rng_seed
  +Noise : Outport
  wires:
  Band-Limited White Noise/1 -> Add2/2
  Signal/1 -> Add2/1
  Add2/1 -> +Noise/1

== system cf_compare_model/PID/Estimator/AddNoise3/AddNoise ==
  Signal : Inport
  Add2 : Sum
  Band-Limited White Noise : simulink/Sources/Band-Limited White Noise  Cov=0.00005  Ts=0.1  seed=rng_seed
  +Noise : Outport
  wires:
  Add2/1 -> +Noise/1
  Signal/1 -> Add2/1
  Band-Limited White Noise/1 -> Add2/2

== system cf_compare_model/PID/Estimator/AddNoise3/AddNoise1 ==
  Signal : Inport
  Add2 : Sum
  Band-Limited White Noise : simulink/Sources/Band-Limited White Noise  Cov=0.00005  Ts=0.1  seed=rng_seed
  +Noise : Outport
  wires:
  Band-Limited White Noise/1 -> Add2/2
  Signal/1 -> Add2/1
  Add2/1 -> +Noise/1

== system cf_compare_model/PID/Estimator/AddNoise3/AddNoise2 ==
  Signal : Inport
  Add2 : Sum
  Band-Limited White Noise : simulink/Sources/Band-Limited White Noise  Cov=0.00005  Ts=0.1  seed=rng_seed
  +Noise : Outport
  wires:
  Add2/1 -> +Noise/1
  Signal/1 -> Add2/1
  Band-Limited White Noise/1 -> Add2/2

== system cf_compare_model/PID/PID Controller/Attitude Control/PID ==
  Desired : Inport
  Measured : Inport  Port=2
  Add : Sum  Inputs=3
  Derivative : Derivative
  Integrator Limited : Integrator  LimitOutput=on  UpperSaturationLimit=intSat(2,1)  LowerSaturationLimit=-intSat(2,1)
  Kd : Gain  Gain=att(1,3)  OutMin=[-200]  OutMax=[200]
  Ki : Gain  Gain=att(1,2)  OutMin=[-200]  OutMax=[200]
  Kp : Gain  Gain=att(1,1)  OutMin=[-200]  OutMax=[200]
  Subtract : Sum  Inputs=+-
  Output : Outport
  wires:
  Measured/1 -> Subtract/2
  Desired/1 -> Subtract/1
  Ki/1 -> Add/2
  Add/1 -> Output/1
  Kp/1 -> Add/1
  Kd/1 -> Add/3
  Subtract/1 -> Kp/1, Integrator Limited/1, Derivative/1
  Integrator Limited/1 -> Ki/1
  Derivative/1 -> Kd/1

== system cf_compare_model/PID/PID Controller/Attitude Control/PID1 ==
  Desired : Inport
  Measured : Inport  Port=2
  Add : Sum  Inputs=3
  Derivative : Derivative
  Integrator Limited1 : Integrator  LimitOutput=on  UpperSaturationLimit=intSat(2,2)  LowerSaturationLimit=-intSat(2,2)
  Kd : Gain  Gain=att(2,3)  OutMin=[-200]  OutMax=[200]
  Ki : Gain  Gain=att(2,2)  OutMin=[-200]  OutMax=[200]
  Kp : Gain  Gain=att(2,1)  OutMin=[-200]  OutMax=[200]
  Subtract : Sum  Inputs=+-
  Output : Outport
  wires:
  Derivative/1 -> Kd/1
  Integrator Limited1/1 -> Ki/1
  Subtract/1 -> Integrator Limited1/1, Derivative/1, Kp/1
  Kd/1 -> Add/3
  Kp/1 -> Add/1
  Add/1 -> Output/1
  Ki/1 -> Add/2
  Desired/1 -> Subtract/1
  Measured/1 -> Subtract/2

== system cf_compare_model/PID/PID Controller/Attitude Control/PID2 ==
  Desired : Inport
  Measured : Inport  Port=2
  Add : Sum  Inputs=3
  Derivative : Derivative
  Integrator Limited : Integrator  LimitOutput=on  UpperSaturationLimit=intSat(2,3)  LowerSaturationLimit=-intSat(2,3)
  Kd : Gain  Gain=att(3,3)  OutMin=[-200]  OutMax=[200]
  Ki : Gain  Gain=att(3,2)  OutMin=[-200]  OutMax=[200]
  Kp : Gain  Gain=att(3,1)  OutMin=[-200]  OutMax=[200]
  Subtract : Sum  Inputs=+-
  Output : Outport
  wires:
  Measured/1 -> Subtract/2
  Desired/1 -> Subtract/1
  Ki/1 -> Add/2
  Add/1 -> Output/1
  Kp/1 -> Add/1
  Kd/1 -> Add/3
  Subtract/1 -> Kp/1, Integrator Limited/1, Derivative/1
  Integrator Limited/1 -> Ki/1
  Derivative/1 -> Kd/1

== system cf_compare_model/PID/PID Controller/Linear Velocity Control/PID ==
  Desired : Inport
  Measured : Inport  Port=2
  Add : Sum  Inputs=3
  Derivative : Derivative
  Integrator Limited : Integrator  LimitOutput=on  UpperSaturationLimit=intSat(1,1)  LowerSaturationLimit=-intSat(1,1)
  Kd : Gain  Gain=pos(1,3)  OutMin=[-200]  OutMax=[200]
  Ki : Gain  Gain=pos(1,2)  OutMin=[-200]  OutMax=[200]
  Kp : Gain  Gain=pos(1,1)  OutMin=[-200]  OutMax=[200]
  Subtract : Sum  Inputs=+-
  Output : Outport
  wires:
  Measured/1 -> Subtract/2
  Desired/1 -> Subtract/1
  Ki/1 -> Add/2
  Add/1 -> Output/1
  Kp/1 -> Add/1
  Kd/1 -> Add/3
  Subtract/1 -> Kp/1, Integrator Limited/1, Derivative/1
  Integrator Limited/1 -> Ki/1
  Derivative/1 -> Kd/1

== system cf_compare_model/PID/PID Controller/Linear Velocity Control/PID1 ==
  Desired : Inport
  Measured : Inport  Port=2
  Add : Sum  Inputs=3
  Derivative : Derivative
  Integrator Limited : Integrator  LimitOutput=on  UpperSaturationLimit=intSat(1,2)  LowerSaturationLimit=-intSat(1,2)
  Kd : Gain  Gain=pos(2,3)  OutMin=[-200]  OutMax=[200]
  Ki : Gain  Gain=pos(2,2)  OutMin=[-200]  OutMax=[200]
  Kp : Gain  Gain=pos(2,1)  OutMin=[-200]  OutMax=[200]
  Subtract : Sum  Inputs=+-
  Output : Outport
  wires:
  Derivative/1 -> Kd/1
  Integrator Limited/1 -> Ki/1
  Subtract/1 -> Derivative/1, Integrator Limited/1, Kp/1
  Kd/1 -> Add/3
  Kp/1 -> Add/1
  Add/1 -> Output/1
  Ki/1 -> Add/2
  Desired/1 -> Subtract/1
  Measured/1 -> Subtract/2

== system cf_compare_model/PID/PID Controller/Linear Velocity Control/PID_Altitude ==
  z_error : Inport
  Add : Sum  Inputs=3
  Derivative : Derivative
  Integrator Limited : Integrator  LimitOutput=on  UpperSaturationLimit=1000  LowerSaturationLimit=-1000
  Kd : Gain  Gain=pos(3,3)  OutMin=[-200]  OutMax=[200]
  Ki : Gain  Gain=pos(3,2)  OutMin=[-200]  OutMax=[200]
  Kp : Gain  Gain=pos(3,1)  OutMin=[-200]  OutMax=[200]
  Adjust : Outport
  wires:
  Derivative/1 -> Kd/1
  Integrator Limited/1 -> Ki/1
  Kd/1 -> Add/3
  Kp/1 -> Add/1
  Ki/1 -> Add/2
  Add/1 -> Adjust/1
  z_error/1 -> Kp/1, Derivative/1, Integrator Limited/1

== system cf_compare_model/PID/PID Controller/Rate Control/PID ==
  Desired : Inport
  Measured : Inport  Port=2
  Add : Sum  Inputs=3
  Derivative : Derivative
  Integrator Limited : Integrator  LimitOutput=on  UpperSaturationLimit=intSat(3,1)  LowerSaturationLimit=-intSat(3,1)
  Kd : Gain  Gain=rates(1,3)  OutMin=[-200]  OutMax=[200]
  Ki : Gain  Gain=rates(1,2)  OutMin=[-200]  OutMax=[200]
  Kp : Gain  Gain=rates(1,1)  OutMin=[-200]  OutMax=[200]
  Subtract : Sum  Inputs=+-
  Output : Outport
  wires:
  Measured/1 -> Subtract/2
  Desired/1 -> Subtract/1
  Ki/1 -> Add/2
  Add/1 -> Output/1
  Kp/1 -> Add/1
  Kd/1 -> Add/3
  Subtract/1 -> Kp/1, Integrator Limited/1, Derivative/1
  Integrator Limited/1 -> Ki/1
  Derivative/1 -> Kd/1

== system cf_compare_model/PID/PID Controller/Rate Control/PID1 ==
  Desired : Inport
  Measured : Inport  Port=2
  Add : Sum  Inputs=3
  Derivative : Derivative
  Integrator Limited : Integrator  LimitOutput=on  UpperSaturationLimit=intSat(3,2)  LowerSaturationLimit=-intSat(3,2)
  Kd : Gain  Gain=rates(2,3)  OutMin=[-200]  OutMax=[200]
  Ki : Gain  Gain=rates(2,2)  OutMin=[-200]  OutMax=[200]
  Kp : Gain  Gain=rates(2,1)  OutMin=[-200]  OutMax=[200]
  Subtract : Sum  Inputs=+-
  Output : Outport
  wires:
  Derivative/1 -> Kd/1
  Integrator Limited/1 -> Ki/1
  Subtract/1 -> Derivative/1, Integrator Limited/1, Kp/1
  Kd/1 -> Add/3
  Kp/1 -> Add/1
  Add/1 -> Output/1
  Ki/1 -> Add/2
  Desired/1 -> Subtract/1
  Measured/1 -> Subtract/2

== system cf_compare_model/PID/PID Controller/Rate Control/PID2 ==
  Desired : Inport
  Measured : Inport  Port=2
  Add : Sum  Inputs=3
  Derivative : Derivative
  Integrator Limited : Integrator  LimitOutput=on  UpperSaturationLimit=intSat(3,3)  LowerSaturationLimit=-intSat(3,3)
  Kd : Gain  Gain=rates(3,3)  OutMin=[-200]  OutMax=[200]
  Ki : Gain  Gain=rates(3,2)  OutMin=[-200]  OutMax=[200]
  Kp : Gain  Gain=rates(3,1)  OutMin=[-200]  OutMax=[200]
  Subtract : Sum  Inputs=+-
  Output : Outport
  wires:
  Measured/1 -> Subtract/2
  Desired/1 -> Subtract/1
  Ki/1 -> Add/2
  Add/1 -> Output/1
  Kp/1 -> Add/1
  Kd/1 -> Add/3
  Subtract/1 -> Kp/1, Integrator Limited/1, Derivative/1
  Integrator Limited/1 -> Ki/1
  Derivative/1 -> Kd/1

== matlab function cf_compare_model/PID/Vehicle/Vehicle Dynamics/MATLAB Function ==
  data: uvw input; xyz_dot output; angles input
function xyz_dot  = Position(uvw,angles)
xyz_dot = zeros(3,1);
phi = angles(1); %*pi/180;
theta = angles(2); %*pi/180;
psi = angles(3); %*pi/180;
Tb_o = [cos(theta)*cos(psi)                                cos(theta)*sin(psi)                             -sin(theta)  ;   %BBF > Inertial rotation matrix
        sin(phi)*sin(theta)*cos(psi)-cos(phi)*sin(psi)    sin(phi)*sin(theta)*sin(psi)+cos(phi)*cos(psi)  sin(phi)*cos(theta) ;
        cos(phi)*sin(theta)*cos(psi)+sin(phi)*sin(psi)    cos(phi)*sin(theta)*sin(psi)-sin(phi)*cos(psi)   cos(phi)*cos(theta)];

xyz_dot = (Tb_o')*uvw;
end

== matlab function cf_compare_model/PID/PID Controller/MATLAB Function1 ==
  data: position input; position_error output; desired_position input
function position_error  = world_error(position,desired_position)
%#Position Error in world Frame
position_error = [0;0;0];


position_error = [desired_position(1)-position(1);...
                  desired_position(2)-position(2);...
                  desired_position(3)-position(3)];

end

== matlab function cf_compare_model/PID/Vehicle/Vehicle Dynamics/MATLAB Function1 ==
  data: pqr input; angles_dot output; angles input
function angles_dot  = Angle(pqr,angles)
angles_dot = zeros(3,1);
phi = angles(1); %*pi/180;
theta = angles(2); %*pi/180;

H = [1    sin(phi)*tan(theta)     cos(phi)*tan(theta)
     0       cos(phi)                 -sin(phi)   
     0       sin(phi)/cos(theta)    cos(phi)/cos(theta)];
angles_dot = H*pqr;
end

== matlab function cf_compare_model/circle yz /Calc_Omg_des  ==
  data: a_des input; omg_des output; j_des input; s_des input; yaw_des input; dyaw_des input; ddyaw_des input; omg_des_dot output
function [omg_des, omg_des_dot]= fcn(a_des, j_des, s_des, yaw_des, dyaw_des, ddyaw_des)
thrust = a_des+[0 0 9.81]';
u1_m = norm(thrust);
z_b = thrust/u1_m;
x_w = [cos(yaw_des) sin(yaw_des) 0];
y_b = cross(z_b, x_w);
y_b = y_b/norm(y_b);
x_b = cross(y_b, z_b);

u1_dot_m = dot(z_b, j_des);
h_w = (j_des - u1_dot_m*z_b)/u1_m;

p = -dot(h_w, y_b);
q = dot(h_w, x_b);
r = dyaw_des*z_b(3);
omg_des = [p q r]';

u1_ddot_m = dot(z_b, s_des) - dot(z_b, cross(omg_des, cross(omg_des, u1_m*z_b)));
h_a = (s_des - u1_ddot_m*z_b - 2*cross(omg_des, u1_dot_m*z_b) - cross(omg_des, cross(omg_des, u1_m*z_b)))/u1_m;

p_dot = -dot(h_a, y_b);
q_dot = dot(h_a, x_b);
r_dot = ddyaw_des*z_b(3);
omg_des_dot = [p_dot, q_dot, r_dot]';

== matlab function cf_compare_model/PID/Vehicle/Vehicle Dynamics/MATLAB Function2 ==
  data: uvw input; uvw_dot output; pqr input; angles input; F input; model parameter
function uvw_dot  = Forces(uvw,pqr,angles,F,model)
uvw_dot = zeros(3,1);
drag = -uvw .* model.c_drag .* model.AirDensity .* model.a;

Force = [0;0;F]+drag;
g_o = [0;0;-9.81];

phi = angles(1); %*pi/180;
theta = angles(2); %*pi/180;
psi = angles(3); %*pi/180;
Tb_o = [cos(theta)*cos(psi)                                cos(theta)*sin(psi)                             -sin(theta)  ;   %BBF > Inertial rotation matrix
        sin(phi)*sin(theta)*cos(psi)-cos(phi)*sin(psi)    sin(phi)*sin(theta)*sin(psi)+cos(phi)*cos(psi)  sin(phi)*cos(theta) ;
        cos(phi)*sin(theta)*cos(psi)+sin(phi)*sin(psi)    cos(phi)*sin(theta)*sin(psi)-sin(phi)*cos(psi)   cos(phi)*cos(theta)];

uvw_dot = Force + Tb_o*g_o - cross(pqr,uvw);
 
end

== matlab function cf_compare_model/PID/Vehicle/Vehicle Dynamics/MATLAB Function3 ==
  data: pqr_dot output; pqr input; M input
function pqr_dot  = Moments(pqr,M)
pqr_dot = zeros(3,1);
Ixx =  1.395e-05;  %2.3951e-5; %1.39e-05; %2.51943e-5; % % %
Iyy = 1.436e-05; %2.3951e-5; %1.436e-05; % 2.54379e-5; % %         %
Izz =  2.173e-05;  %3.2347e-5; %2.173e-05 ; %4.51407e-5; % %         %;%0.160;
J = diag([Ixx Iyy Izz]);    %   I  Flyer rotational inertia matrix     3x3
pqr_dot = inv(J)*(M-cross(pqr,J*pqr));
end

== matlab function cf_compare_model/PID/Estimator/Mahoney/calc v3 ==
  data: q input; v output
function v = fcn(q)
%#codegen
v = zeros(3,1);
v = [2*(q(2)*q(4) - q(1)*q(3))
         2*(q(1)*q(2) + q(3)*q(4))
         q(1)^2 - q(2)^2 - q(3)^2 + q(4)^2];
end

== matlab function cf_compare_model/PID/Estimator/Mahoney/calc v ==
  data: q input; v output
function v = fcn(q)
%#codegen
v = zeros(3,1);
v = [2*(q(2)*q(4) - q(1)*q(3))
         2*(q(1)*q(2) + q(3)*q(4))
         q(1)^2 - q(2)^2 - q(3)^2 + q(4)^2];
end

== matlab function cf_compare_model/PID/Estimator/Mahoney/quatprod ==
  data: a input; ab output; b input
function ab = quaternProd(a, b)
%QUATERNPROD Calculates the quaternion product
%
%   ab = quaternProd(a, b)
%
%   Calculates the quaternion product of quaternion a and b.
%
%   For more information see:
%   http://www.x-io.co.uk/node/8#quaternions
%
%	Date          Author          Notes
%	27/09/2011    SOH Madgwick    Initial release
    ab = zeros(1,4);
    ab(:,1) = a(:,1).*b(:,1)-a(:,2).*b(:,2)-a(:,3).*b(:,3)-a(:,4).*b(:,4);
    ab(:,2) = a(:,1).*b(:,2)+a(:,2).*b(:,1)+a(:,3).*b(:,4)-a(:,4).*b(:,3);
    ab(:,3) = a(:,1).*b(:,3)-a(:,2).*b(:,4)+a(:,3).*b(:,1)+a(:,4).*b(:,2);
    ab(:,4) = a(:,1).*b(:,4)+a(:,2).*b(:,3)-a(:,3).*b(:,2)+a(:,4).*b(:,1);
end

== matlab function cf_compare_model/PID Controller/MATLAB Function1 ==
  data: position input; position_error output; desired_position input
function position_error  = world_error(position,desired_position)
%#Position Error in world Frame
position_error = [0;0;0];


position_error = [desired_position(1)-position(1);...
                  desired_position(2)-position(2);...
                  desired_position(3)-position(3)];

end

== matlab function cf_compare_model/PID_Estimator/Mahony/calc v ==
  data: q input; v output
function v = fcn(q)
%#codegen
v = zeros(3,1);
v = [2*(q(2)*q(4) - q(1)*q(3))
         2*(q(1)*q(2) + q(3)*q(4))
         q(1)^2 - q(2)^2 - q(3)^2 + q(4)^2];
end

== matlab function cf_compare_model/PID_Estimator/Mahony/calc v3 ==
  data: q input; v output
function v = fcn(q)
%#codegen
v = zeros(3,1);
v = [2*(q(2)*q(4) - q(1)*q(3))
         2*(q(1)*q(2) + q(3)*q(4))
         q(1)^2 - q(2)^2 - q(3)^2 + q(4)^2];
end

== matlab function cf_compare_model/PID_Estimator/Mahony/quatprod ==
  data: a input; ab output; b input
function ab = quaternProd(a, b)
%QUATERNPROD Calculates the quaternion product
%
%   ab = quaternProd(a, b)
%
%   Calculates the quaternion product of quaternion a and b.
%
%   For more information see:
%   http://www.x-io.co.uk/node/8#quaternions
%
%	Date          Author          Notes
%	27/09/2011    SOH Madgwick    Initial release
    ab = zeros(1,4);
    ab(:,1) = a(:,1).*b(:,1)-a(:,2).*b(:,2)-a(:,3).*b(:,3)-a(:,4).*b(:,4);
    ab(:,2) = a(:,1).*b(:,2)+a(:,2).*b(:,1)+a(:,3).*b(:,4)-a(:,4).*b(:,3);
    ab(:,3) = a(:,1).*b(:,3)-a(:,2).*b(:,4)+a(:,3).*b(:,1)+a(:,4).*b(:,2);
    ab(:,4) = a(:,1).*b(:,4)+a(:,2).*b(:,3)-a(:,3).*b(:,2)+a(:,4).*b(:,1);
end

== matlab function cf_compare_model/GC_Estimator/Mahony/calc v ==
  data: q input; v output
function v = fcn(q)
%#codegen
v = zeros(3,1);
v = [2*(q(2)*q(4) - q(1)*q(3))
         2*(q(1)*q(2) + q(3)*q(4))
         q(1)^2 - q(2)^2 - q(3)^2 + q(4)^2];
end

== matlab function cf_compare_model/Vehicle1/Vehicle Dynamics/MATLAB Function ==
  data: uvw input; xyz_dot output; angles input
function xyz_dot  = Position(uvw,angles)
xyz_dot = zeros(3,1);
phi = angles(1); %*pi/180;
theta = angles(2); %*pi/180;
psi = angles(3); %*pi/180;
Tb_o = [cos(theta)*cos(psi)                                cos(theta)*sin(psi)                             -sin(theta)  ;   %BBF > Inertial rotation matrix
        sin(phi)*sin(theta)*cos(psi)-cos(phi)*sin(psi)    sin(phi)*sin(theta)*sin(psi)+cos(phi)*cos(psi)  sin(phi)*cos(theta) ;
        cos(phi)*sin(theta)*cos(psi)+sin(phi)*sin(psi)    cos(phi)*sin(theta)*sin(psi)-sin(phi)*cos(psi)   cos(phi)*cos(theta)];

xyz_dot = (Tb_o')*uvw;
end

== matlab function cf_compare_model/GC_Estimator/Mahony/calc v3 ==
  data: q input; v output
function v = fcn(q)
%#codegen
v = zeros(3,1);
v = [2*(q(2)*q(4) - q(1)*q(3))
         2*(q(1)*q(2) + q(3)*q(4))
         q(1)^2 - q(2)^2 - q(3)^2 + q(4)^2];
end

== matlab function cf_compare_model/Vehicle1/Vehicle Dynamics/MATLAB Function1 ==
  data: pqr input; angles_dot output; angles input
function angles_dot  = Angle(pqr,angles)
angles_dot = zeros(3,1);
phi = angles(1); %*pi/180;
theta = angles(2); %*pi/180;

H = [1    sin(phi)*tan(theta)     cos(phi)*tan(theta)
     0       cos(phi)                 -sin(phi)   
     0       sin(phi)/cos(theta)    cos(phi)/cos(theta)];
angles_dot = H*pqr;
end

== matlab function cf_compare_model/Vehicle1/Vehicle Dynamics/MATLAB Function2 ==
  data: uvw input; uvw_dot output; pqr input; angles input; F input
function uvw_dot  = Forces(uvw,pqr,angles,F)
uvw_dot = zeros(3,1);
Force = [0;0;F];
g_o = [0;0;-9.81];
phi = angles(1); %*pi/180;
theta = angles(2); %*pi/180;
psi = angles(3); %*pi/180;
Tb_o = [cos(theta)*cos(psi)                                cos(theta)*sin(psi)                             -sin(theta)  ;   %BBF > Inertial rotation matrix
        sin(phi)*sin(theta)*cos(psi)-cos(phi)*sin(psi)    sin(phi)*sin(theta)*sin(psi)+cos(phi)*cos(psi)  sin(phi)*cos(theta) ;
        cos(phi)*sin(theta)*cos(psi)+sin(phi)*sin(psi)    cos(phi)*sin(theta)*sin(psi)-sin(phi)*cos(psi)   cos(phi)*cos(theta)];

uvw_dot = Force + Tb_o*g_o - cross(pqr,uvw);

end

== matlab function cf_compare_model/Vehicle1/Vehicle Dynamics/MATLAB Function3 ==
  data: pqr_dot output; pqr input; M input
function pqr_dot  = Moments(pqr,M)
pqr_dot = zeros(3,1);
Ixx =  1.395e-05;  %2.3951e-5; %1.39e-05; %2.51943e-5; % % %
Iyy = 1.436e-05; %2.3951e-5; %1.436e-05; % 2.54379e-5; % %         %
Izz =  2.173e-05;  %3.2347e-5; %2.173e-05 ; %4.51407e-5; % %         %;%0.160;
J = diag([Ixx Iyy Izz]);    %   I  Flyer rotational inertia matrix     3x3
pqr_dot = inv(J)*(M-cross(pqr,J*pqr));
end

== matlab function cf_compare_model/GC_Estimator/Mahony/quatprod ==
  data: a input; ab output; b input
function ab = quaternProd(a, b)
%QUATERNPROD Calculates the quaternion product
%
%   ab = quaternProd(a, b)
%
%   Calculates the quaternion product of quaternion a and b.
%
%   For more information see:
%   http://www.x-io.co.uk/node/8#quaternions
%
%	Date          Author          Notes
%	27/09/2011    SOH Madgwick    Initial release
    ab = zeros(1,4);
    ab(:,1) = a(:,1).*b(:,1)-a(:,2).*b(:,2)-a(:,3).*b(:,3)-a(:,4).*b(:,4);
    ab(:,2) = a(:,1).*b(:,2)+a(:,2).*b(:,1)+a(:,3).*b(:,4)-a(:,4).*b(:,3);
    ab(:,3) = a(:,1).*b(:,3)-a(:,2).*b(:,4)+a(:,3).*b(:,1)+a(:,4).*b(:,2);
    ab(:,4) = a(:,1).*b(:,4)+a(:,2).*b(:,3)-a(:,3).*b(:,2)+a(:,4).*b(:,1);
end

== matlab function cf_compare_model/circle xy/Calc_Omg_des  ==
  data: a_des input; omg_des output; j_des input; s_des input; yaw_des input; dyaw_des input; ddyaw_des input; omg_des_dot output
function [omg_des, omg_des_dot]= fcn(a_des, j_des, s_des, yaw_des, dyaw_des, ddyaw_des)
thrust = a_des+[0 0 9.81]';
u1_m = norm(thrust);
z_b = thrust/u1_m;
x_w = [cos(yaw_des) sin(yaw_des) 0];
y_b = cross(z_b, x_w);
y_b = y_b/norm(y_b);
x_b = cross(y_b, z_b);

u1_dot_m = dot(z_b, j_des);
h_w = (j_des - u1_dot_m*z_b)/u1_m;

p = -dot(h_w, y_b);
q = dot(h_w, x_b);
r = dyaw_des*z_b(3);
omg_des = [p q r]';

u1_ddot_m = dot(z_b, s_des) - dot(z_b, cross(omg_des, cross(omg_des, u1_m*z_b)));
h_a = (s_des - u1_ddot_m*z_b - 2*cross(omg_des, u1_dot_m*z_b) - cross(omg_des, cross(omg_des, u1_m*z_b)))/u1_m;

p_dot = -dot(h_a, y_b);
q_dot = dot(h_a, x_b);
r_dot = ddyaw_des*z_b(3);
omg_des_dot = [p_dot, q_dot, r_dot]';

== matlab function cf_compare_model/Vehicle3/Vehicle Dynamics/MATLAB Function ==
  data: uvw input; xyz_dot output; angles input
function xyz_dot  = Position(uvw,angles)
xyz_dot = zeros(3,1);
phi = angles(1); %*pi/180;
theta = angles(2); %*pi/180;
psi = angles(3); %*pi/180;
Tb_o = [cos(theta)*cos(psi)                                cos(theta)*sin(psi)                             -sin(theta)  ;   %BBF > Inertial rotation matrix
        sin(phi)*sin(theta)*cos(psi)-cos(phi)*sin(psi)    sin(phi)*sin(theta)*sin(psi)+cos(phi)*cos(psi)  sin(phi)*cos(theta) ;
        cos(phi)*sin(theta)*cos(psi)+sin(phi)*sin(psi)    cos(phi)*sin(theta)*sin(psi)-sin(phi)*cos(psi)   cos(phi)*cos(theta)];

xyz_dot = (Tb_o')*uvw;
end

== matlab function cf_compare_model/Vehicle3/Vehicle Dynamics/MATLAB Function1 ==
  data: pqr input; angles_dot output; angles input
function angles_dot  = Angle(pqr,angles)
angles_dot = zeros(3,1);
phi = angles(1); %*pi/180;
theta = angles(2); %*pi/180;

H = [1    sin(phi)*tan(theta)     cos(phi)*tan(theta)
     0       cos(phi)                 -sin(phi)   
     0       sin(phi)/cos(theta)    cos(phi)/cos(theta)];
angles_dot = H*pqr;
end

== matlab function cf_compare_model/Vehicle3/Vehicle Dynamics/MATLAB Function2 ==
  data: uvw input; uvw_dot output; pqr input; angles input; F input
function uvw_dot  = Forces(uvw,pqr,angles,F)
uvw_dot = zeros(3,1);
Force = [0;0;F];
g_o = [0;0;-9.81];
phi = angles(1); %*pi/180;
theta = angles(2); %*pi/180;
psi = angles(3); %*pi/180;
Tb_o = [cos(theta)*cos(psi)                                cos(theta)*sin(psi)                             -sin(theta)  ;   %BBF > Inertial rotation matrix
        sin(phi)*sin(theta)*cos(psi)-cos(phi)*sin(psi)    sin(phi)*sin(theta)*sin(psi)+cos(phi)*cos(psi)  sin(phi)*cos(theta) ;
        cos(phi)*sin(theta)*cos(psi)+sin(phi)*sin(psi)    cos(phi)*sin(theta)*sin(psi)-sin(phi)*cos(psi)   cos(phi)*cos(theta)];

uvw_dot = Force + Tb_o*g_o - cross(pqr,uvw);

end

== matlab function cf_compare_model/Vehicle3/Vehicle Dynamics/MATLAB Function3 ==
  data: pqr_dot output; pqr input; M input
function pqr_dot  = Moments(pqr,M)
pqr_dot = zeros(3,1);
Ixx =  1.395e-05;  %2.3951e-5; %1.39e-05; %2.51943e-5; % % %
Iyy = 1.436e-05; %2.3951e-5; %1.436e-05; % 2.54379e-5; % %         %
Izz =  2.173e-05;  %3.2347e-5; %2.173e-05 ; %4.51407e-5; % %         %;%0.160;
J = diag([Ixx Iyy Izz]);    %   I  Flyer rotational inertia matrix     3x3
pqr_dot = inv(J)*(M-cross(pqr,J*pqr));
end
